simulink model "lab2"  (R2017b)
settings: Solver=ode4  StartTime=0.0  StopTime=10.0  FixedStep=0.0001  RelTol=1e-3
settings Model: Creator=ayushi  LastModifiedBy=ayushi

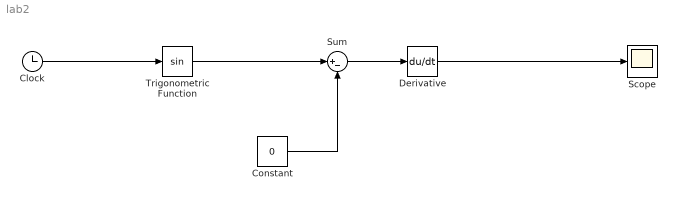
== system lab2 ==
  Clock : Clock
  Constant : Constant  Value=0
  Derivative : Derivative
  Scope : Scope
  Sum : Sum  Inputs=|+-
  Trigonometric Function : Trigonometry
  wires:
  Clock/1 -> Trigonometric Function/1
  Trigonometric Function/1 -> Sum/1
  Constant/1 -> Sum/2
  Sum/1 -> Derivative/1
  Derivative/1 -> Scope/1
